simulink model "DSSDK_TrackerSingleObject"  (Simulink 9.3)
settings: Solver=FixedStepDiscrete  StartTime=0.0  StopTime=inf  FixedStep=Ts  RelTol=1e-3  EnableMultiTasking=on
StopFcn:
  | save('viconData.mat','viconData')
undefined symbols (not defined in the file or in its folder): fdesignblkfcn, gcbh
libraries: simulink x5, parrotlib x2
settings Model: Creator=Ssubrama  LastModifiedBy=yahyaaba
settings DataIOCC: LimitDataPoints=on
settings OptimizationCC: ExpressionDepthLimit=2147483647  InitFltsAndDblsToZero=on
settings DebuggingCC: SolverPrmCheckMsg=warning  StateNameClashWarn=warning
settings GRTTargetCC: TargetFcnLib=ansi_tfl_tmw_new.mat  GeneratePreprocessorConditionals=Disable all
settings ConfigComp: CovSFcnEnable=off

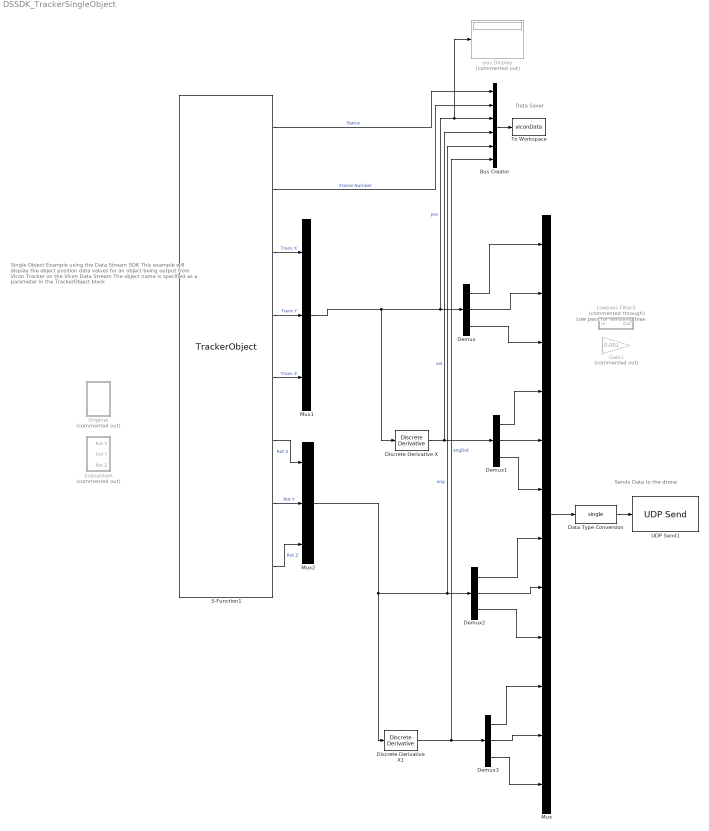
== system DSSDK_TrackerSingleObject ==
  note: Sends Data to the drone
  note: Data Saver
  note: Low pass for removing bias
  note: Single Object Example
      | using the Data Stream SDK
      |
      | This example will display the object position data
      | values for an object being output from
      | Vicon Tracker on the Vicon Data Stream
      |
      | The object name is specified as a parameter
      | in the TrackerObject block
  Bus Creator : BusCreator  Inputs=6
  Data Type Conversion : DataTypeConversion  OutDataTypeStr=single
  Demux{,1..3} (4 alike) : Demux  Outputs=3
  Discrete Derivative X : simulink/Discrete/Discrete Derivative  gainval=1.0  ICPrevScaledInput=0.0  OutMin=[]  OutMax=[]  OutDataType=fixdt(1, 16)  OutScaling=2^-10  DoSatur=off
  Discrete Derivative X1 : simulink/Discrete/Discrete Derivative  gainval=1.0  ICPrevScaledInput=0.0  OutMin=[]  OutMax=[]  OutDataType=fixdt(1, 16)  OutScaling=2^-10  DoSatur=off
  Gain1 : Gain  Commented=on  Gain=0.001
  Lowpass Filter3 : Subsystem  Commented=through  DialogController=fdesignblkfcn  DialogControllerArgs=DataTag1  InitFcn=fdesignblkfcn(gcbh, {'InitFcn'});  mask(Lowpass Filter){}
      mask help: Design a lowpass filter
      settings: CopyFcn=fdesignblkfcn(gcbh, {'CopyFcn'});
      mask Help: helpview(mapfilelocation('dsp'), 'dsplowpassfilter');
      mask Display: disp('Lowpass')
  Mux : Mux  Inputs=12
  Mux1 : Mux  Inputs=3
  Mux2 : Mux  Inputs=3
  Original : Subsystem  Commented=on
  S-Function1 : S-Function  FunctionName=TrackerObject  Parameters='ParrotMambo'  SFunctionModules=TrackerObject  SFunctionDeploymentMode=off  EnableBusSupport=off
      settings: AttributesFormatString=Data Parser
  Subsystem : Subsystem  Commented=on
  To Workspace : ToWorkspace  VariableName=viconData  SaveFormat=Timeseries  SampleTime=-1
  UDP Send1 : parrotlib/UDP Send  remoteURL='192.168.3.1'  remotePort=25000  localURL='0.0.0.0'  localPortSource=Automatically determine  localPort=2048  sampletime=-1  blockPlatform=LINUX  separateLengthPort=0
      settings: SourceProductName=Simulink Support Package for PARROT Minidrones  SourceProductBaseCode=MINIDRONES
  pos Display : Display  Commented=on
  wires:
  S-Function1/3 -> Mux1/1  "Trans X"
  S-Function1/5 -> Mux1/3  "Trans Z"
  Data Type Conversion/1 -> UDP Send1/1
  Mux/1 -> Data Type Conversion/1
  S-Function1/6 -> Mux2/1  "Rot X"
  S-Function1/7 -> Mux2/2  "Rot Y"
  S-Function1/8 -> Mux2/3  "Rot Z"
  S-Function1/1 -> Bus Creator/1  "Status"
  S-Function1/2 -> Bus Creator/2  "Frame Number"
  S-Function1/4 -> Mux1/2  "Trans Y"
  Mux1/1 -> pos Display/1, Bus Creator/3, Demux/1, Discrete Derivative X/1  "pos"
  Demux/1 -> Mux/1
  Demux/2 -> Mux/2
  Demux/3 -> Mux/3
  Demux1/1 -> Mux/4
  Demux1/2 -> Mux/5
  Demux1/3 -> Mux/6
  Demux2/1 -> Mux/7
  Demux2/2 -> Mux/8
  Demux2/3 -> Mux/9
  Discrete Derivative X1/1 -> Demux3/1, Bus Creator/6  "angDot"
  Demux3/1 -> Mux/10
  Demux3/2 -> Mux/11
  Demux3/3 -> Mux/12
  Mux2/1 -> Demux2/1, Bus Creator/5, Discrete Derivative X1/1  "ang"
  Discrete Derivative X/1 -> Bus Creator/4, Demux1/1  "vel"
  Bus Creator/1 -> To Workspace/1

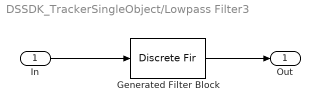
== system DSSDK_TrackerSingleObject/Lowpass Filter3 ==
  In : Inport
  Generated Filter Block : DiscreteFir  Tag=BlockMethodSubSystem  Coefficients=[0.00055930462501575318 0.000134387355635492544 0.000150164544220283578 0.000166938571918249026 0.000184913426126165478 0.000204159638341897876 0.000224847539957342317 0.000246888557047488118 0.000270250930713089371 0.000294678714756113928 0.000320320592567133189 0.000347381610550177703 0.000376503237496001526 0.000407063236803795311 0.000437969836956363285 0.000471966634088865277 0.000506629618629239609 0.000543258400010798704 0.000581446667477806102 0.000621483478831086908 0.000663240114968196475 0.000706786791731873467 0.000751966629339840078 0.000798957232007100585 0.000847786970567231948 0.000898567434806632503 0.000950986800426248521 0.00100536098241037187 0.00106189549677395854 0.00111999258611391694 0.00118025266269442377 0.00124231961860752629 0.00130642002474549318 0.00137244110948316739 0.00144041400814671496 0.00151028782591035434 0.00158214490911966644 0.00165593031316057463 0.00173161625085798245 0.00180913894205901355 0.00188869079631055563 0.00197008991505943183 0.00205326044396706353 0.00213839755526306231 0.00222523410058983809 0.0023139366140836953 0.00240433500877287442 0.00249647034146493986 0.00259028150327670834 0.00268577672918223105 0.00278284271081329342 0.00288145055032864748 0.00298156134317205564 0.00308318312494121945 0.0031861164566033065 0.00329041971903219245 0.00339602350822430007 0.00350278519574314436 0.00361074370565326631 0.00371971960476352465 0.00382972885080347814 0.00394066786669221118 0.00405247698115740549 0.00416504159927491568 0.00427831667671187306 0.00439222319691515498 0.00450666349417792877 0.00462150504328727105 0.00473675818605371994 0.0048522536812996564 0.00496792387820703223 0.00508369550725730566 0.00519941524626886878 0.00531505864840853791 0.00543047442906128414 0.00554558136902359722 0.00566026462488985246 0.00577445307225213627 0.00588802605681441188 0.00600086635173012646 0.00611287829882902096 0.00622399830399815272 0.00633405571686646452 0.00644301018993313247 0.00655072347056720461 0.00665709789858928702 0.00676205989040209836 0.00686546177223198301 0.00696722908918023624 0.00706725534584395215 0.00716545349111825242 0.00726170727371388321 0.00735591743291842421 0.00744801050560451022 0.00753788345848689558 0.0076254188763999961 0.00771057173373233817 0.00779320792465807571 0.00787327807504492778 0.00795068643545090992 0.00802533165362758101 0.00809716296896351162 0.00816609203546844568 0.00823205161182060871 0.00829495997208222306 0.00835475861758848935 0.00841139903382095468 0.00846479300015721449 0.00851489303009545818 0.0085616579958750251 0.00860500810577487923 0.0086449345827915719 0.00868135979237836738 0.00871425404479079894 0.00874359520388623412 0.00876933590254826839 0.00879145283398880331 0.00880991471525752537 0.00882471405033441632 0.00883583717884927483 0.0088432445604231108 0.00884695935983879043 0.00884695935983879043 0.0088432445604231108 0.00883583717884927483 0.00882471405033441632 0.00880991471525752537 0.00879145283398880331 0.00876933590254826839 0.00874359520388623412 0.00871425404479079894 0.00868135979237836738 0.0086449345827915719 0.00860500810577487923 0.0085616579958750251 0.00851489303009545818 0.00846479300015721449 0.00841139903382095468 0.00835475861758848935 0.00829495997208222306 0.00823205161182060871 0.00816609203546844568 0.00809716296896351162 0.00802533165362758101 0.00795068643545090992 0.00787327807504492778 0.00779320792465807571 0.00771057173373233817 0.0076254188763999961 0.00753788345848689558 0.00744801050560451022 0.00735591743291842421 0.00726170727371388321 0.00716545349111825242 0.00706725534584395215 0.00696722908918023624 0.00686546177223198301 0.00676205989040209836 0.00665709789858928702 0.00655072347056720461 0.00644301018993313247 0.00633405571686646452 0.00622399830399815272 0.00611287829882902096 0.00600086635173012646 0.00588802605681441188 0.00577445307225213627 0.00566026462488985246 0.00554558136902359722 0.00543047442906128414 0.00531505864840853791 0.00519941524626886878 0.00508369550725730566 ...(+1656 chars)]  InputProcessing=Columns as channels (frame based)
  Out : Outport
  wires:
  Generated Filter Block/1 -> Out/1
  In/1 -> Generated Filter Block/1

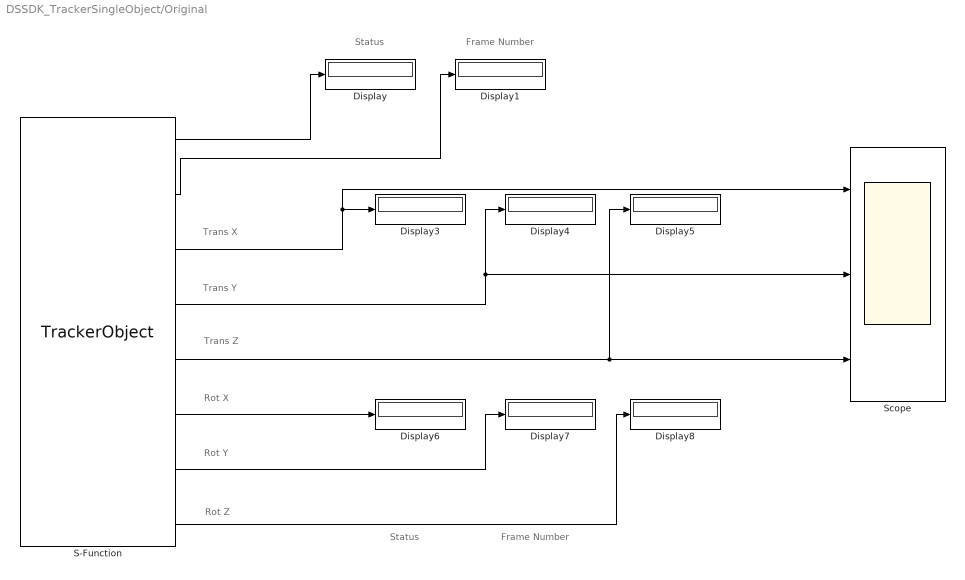
== system DSSDK_TrackerSingleObject/Original ==
  note: Rot Z
  note: Rot Y
  note: Rot X
  note: Trans Z
  note: Trans Y
  note: Trans X
  note: Frame Number
  note: Status
  note: Frame Number
  note: Status
  Display{,1,3..8} (8 alike) : Display
  S-Function : S-Function  FunctionName=TrackerObject  Parameters='Object1'  SFunctionModules=TrackerObject  SFunctionDeploymentMode=off  EnableBusSupport=off
      settings: AttributesFormatString=Data Parser
  Scope : Scope  NumInputPorts=3
  wires:
  S-Function/6 -> Display6/1
  S-Function/7 -> Display7/1
  S-Function/1 -> Display/1
  S-Function/4 -> Display4/1, Scope/2
  S-Function/8 -> Display8/1
  S-Function/5 -> Display5/1, Scope/3
  S-Function/2 -> Display1/1
  S-Function/3 -> Scope/1, Display3/1

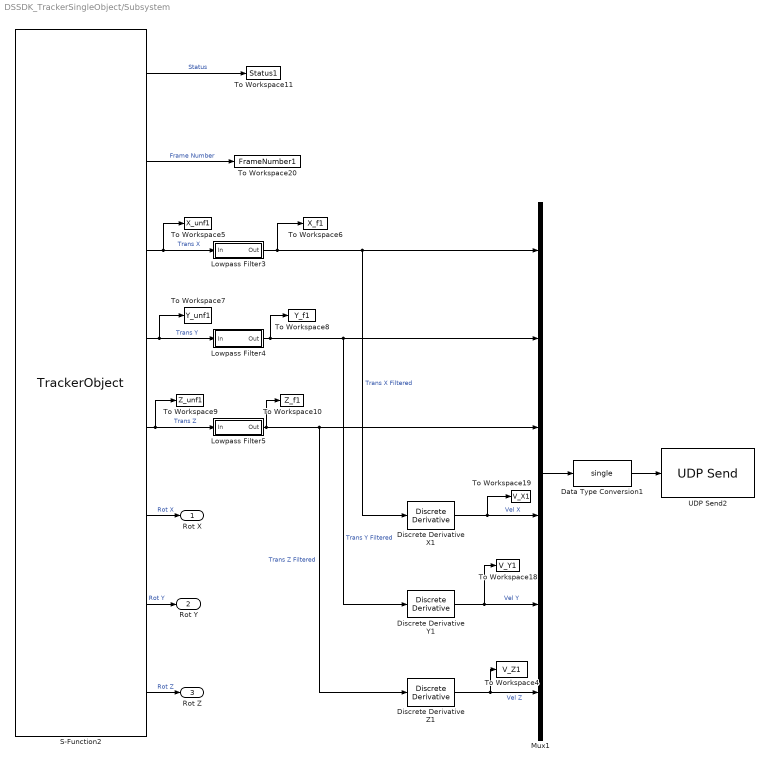
== system DSSDK_TrackerSingleObject/Subsystem ==
  Data Type Conversion1 : DataTypeConversion  OutDataTypeStr=single
  Discrete Derivative X1 : simulink/Discrete/Discrete Derivative  gainval=1.0  ICPrevScaledInput=0.0  OutMin=[]  OutMax=[]  OutDataType=fixdt(1, 16)  OutScaling=2^-10  DoSatur=off
  Discrete Derivative Y1 : simulink/Discrete/Discrete Derivative  gainval=1.0  ICPrevScaledInput=0.0  OutMin=[]  OutMax=[]  OutDataType=fixdt(1, 16)  OutScaling=2^-10  DoSatur=off
  Discrete Derivative Z1 : simulink/Discrete/Discrete Derivative  gainval=1.0  ICPrevScaledInput=0.0  OutMin=[]  OutMax=[]  OutDataType=fixdt(1, 16)  OutScaling=2^-10  DoSatur=off
  Lowpass Filter3 : Subsystem  DialogController=fdesignblkfcn  DialogControllerArgs=DataTag3  InitFcn=fdesignblkfcn(gcbh, {'InitFcn'});  mask(Lowpass Filter){}
      mask help: Design a lowpass filter
      settings: CopyFcn=fdesignblkfcn(gcbh, {'CopyFcn'});
      mask Help: helpview(mapfilelocation('dsp'), 'dsplowpassfilter');
      mask Display: disp('Lowpass')
  Lowpass Filter4 : Subsystem  DialogController=fdesignblkfcn  DialogControllerArgs=DataTag5  InitFcn=fdesignblkfcn(gcbh, {'InitFcn'});  mask(Lowpass Filter){}
      mask help: Design a lowpass filter
      settings: CopyFcn=fdesignblkfcn(gcbh, {'CopyFcn'});
      mask Help: helpview(mapfilelocation('dsp'), 'dsplowpassfilter');
      mask Display: disp('Lowpass')
  Lowpass Filter5 : Subsystem  DialogController=fdesignblkfcn  DialogControllerArgs=DataTag7  InitFcn=fdesignblkfcn(gcbh, {'InitFcn'});  mask(Lowpass Filter){}
      mask help: Design a lowpass filter
      settings: CopyFcn=fdesignblkfcn(gcbh, {'CopyFcn'});
      mask Help: helpview(mapfilelocation('dsp'), 'dsplowpassfilter');
      mask Display: disp('Lowpass')
  Mux1 : Mux  Inputs=6
  S-Function2 : S-Function  FunctionName=TrackerObject  Parameters='Object1'  SFunctionModules=TrackerObject  SFunctionDeploymentMode=off  EnableBusSupport=off
      settings: AttributesFormatString=Data Parser
  To Workspace10 : ToWorkspace  VariableName=Z_f1  SaveFormat=Timeseries  SampleTime=-1
  To Workspace11 : ToWorkspace  VariableName=Status1  SaveFormat=Timeseries  SampleTime=-1
  To Workspace18 : ToWorkspace  VariableName=V_Y1  SaveFormat=Timeseries  SampleTime=-1
  To Workspace19 : ToWorkspace  VariableName=V_X1  SaveFormat=Timeseries  SampleTime=-1
  To Workspace20 : ToWorkspace  VariableName=FrameNumber1  SaveFormat=Timeseries  SampleTime=-1
  To Workspace4 : ToWorkspace  VariableName=V_Z1  SaveFormat=Timeseries  SampleTime=-1
  To Workspace5 : ToWorkspace  VariableName=X_unf1  SaveFormat=Timeseries  SampleTime=-1
  To Workspace6 : ToWorkspace  VariableName=X_f1  SaveFormat=Timeseries  SampleTime=-1
  To Workspace7 : ToWorkspace  VariableName=Y_unf1  SaveFormat=Timeseries  SampleTime=-1
  To Workspace8 : ToWorkspace  VariableName=Y_f1  SaveFormat=Timeseries  SampleTime=-1
  To Workspace9 : ToWorkspace  VariableName=Z_unf1  SaveFormat=Timeseries  SampleTime=-1
  UDP Send2 : parrotlib/UDP Send  remoteURL='192.168.3.1'  remotePort=25000  localURL='0.0.0.0'  localPortSource=Automatically determine  localPort=2048  sampletime=-1  blockPlatform=LINUX  separateLengthPort=0
      settings: SourceProductName=Simulink Support Package for PARROT Minidrones  SourceProductBaseCode=MINIDRONES
  Rot X : Outport
  Rot Y : Outport  Port=2
  Rot Z : Outport  Port=3
  wires:
  S-Function2/7 -> Rot Y/1  "Rot Y"
  Lowpass Filter4/1(Out) -> Discrete Derivative Y1/1, Mux1/2, To Workspace8/1  "Trans Y Filtered"
  Discrete Derivative X1/1 -> Mux1/4, To Workspace19/1  "Vel X"
  S-Function2/5 -> Lowpass Filter5/1(In), To Workspace9/1  "Trans Z"
  S-Function2/4 -> Lowpass Filter4/1(In), To Workspace7/1  "Trans Y"
  S-Function2/2 -> To Workspace20/1  "Frame Number"
  Lowpass Filter5/1(Out) -> To Workspace10/1, Discrete Derivative Z1/1, Mux1/3  "Trans Z Filtered"
  Discrete Derivative Y1/1 -> To Workspace18/1, Mux1/5  "Vel Y"
  S-Function2/1 -> To Workspace11/1  "Status"
  Discrete Derivative Z1/1 -> To Workspace4/1, Mux1/6  "Vel Z"
  Mux1/1 -> Data Type Conversion1/1
  Data Type Conversion1/1 -> UDP Send2/1
  S-Function2/3 -> To Workspace5/1, Lowpass Filter3/1(In)  "Trans X"
  Lowpass Filter3/1(Out) -> Discrete Derivative X1/1, Mux1/1, To Workspace6/1  "Trans X Filtered"
  S-Function2/6 -> Rot X/1  "Rot X"
  S-Function2/8 -> Rot Z/1  "Rot Z"

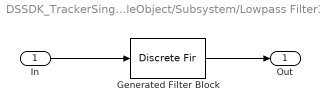
== system DSSDK_TrackerSingleObject/Subsystem/Lowpass Filter3 ==
  In : Inport
  Generated Filter Block : DiscreteFir  Tag=BlockMethodSubSystem  Coefficients=[0.000559304625015753397 0.000134387355635494116 0.000150164544220285801 0.00016693857191824946 0.000184913426126165478 0.00020415963834189831 0.000224847539957342317 0.000246888557047488118 0.000270250930713089588 0.0002946787147561155 0.000320320592567135195 0.000347381610550178842 0.000376503237496001472 0.000407063236803794769 0.000437969836956363719 0.000471966634088866199 0.000506629618629240042 0.000543258400010799571 0.00058144666747780762 0.000621483478831088101 0.000663240114968196908 0.000706786791731873034 0.000751966629339840295 0.000798957232007101669 0.00084778697056723184 0.000898567434806632395 0.000950986800426249172 0.00100536098241037252 0.00106189549677395919 0.00111999258611391803 0.00118025266269442442 0.00124231961860752672 0.00130642002474549426 0.00137244110948316826 0.00144041400814671539 0.00151028782591035478 0.001582144909119666 0.00165593031316057463 0.00173161625085798375 0.00180913894205901441 0.00188869079631055628 0.00197008991505943226 0.00205326044396706439 0.00213839755526306317 0.00222523410058983852 0.0023139366140836953 0.00240433500877287485 0.00249647034146493986 0.00259028150327670877 0.00268577672918223148 0.00278284271081329429 0.00288145055032864791 0.00298156134317205564 0.00308318312494121989 0.0031861164566033065 0.00329041971903219245 0.00339602350822430007 0.00350278519574314436 0.00361074370565326631 0.00371971960476352422 0.00382972885080347814 0.00394066786669221118 0.00405247698115740549 0.00416504159927491568 0.00427831667671187306 0.00439222319691515584 0.00450666349417792877 0.00462150504328727105 0.00473675818605371994 0.0048522536812996564 0.00496792387820703223 0.00508369550725730566 0.00519941524626886878 0.00531505864840853878 0.005430474429061285 0.00554558136902359722 0.00566026462488985246 0.00577445307225213627 0.00588802605681441188 0.00600086635173012646 0.00611287829882902096 0.00622399830399815186 0.00633405571686646365 0.00644301018993313161 0.00655072347056720548 0.00665709789858928702 0.00676205989040209836 0.00686546177223198127 0.00696722908918023538 0.00706725534584395128 0.00716545349111825242 0.00726170727371388321 0.00735591743291842334 0.00744801050560450935 0.00753788345848689471 0.0076254188763999961 0.00771057173373233731 0.00779320792465807398 0.00787327807504492605 0.00795068643545090818 0.00802533165362757928 0.00809716296896350989 0.00816609203546844395 0.00823205161182060698 0.00829495997208222133 0.00835475861758848762 0.00841139903382095294 0.00846479300015721275 0.00851489303009545818 0.0085616579958750251 0.00860500810577487923 0.0086449345827915719 0.00868135979237836738 0.00871425404479079721 0.00874359520388623065 0.00876933590254826839 0.00879145283398879984 0.00880991471525751843 0.00882471405033441458 0.00883583717884927136 0.00884324456042310733 0.0088469593598387887 0.0088469593598387887 0.00884324456042310733 0.00883583717884927136 0.00882471405033441458 0.00880991471525751843 0.00879145283398879984 0.00876933590254826839 0.00874359520388623065 0.00871425404479079721 0.00868135979237836738 0.0086449345827915719 0.00860500810577487923 0.0085616579958750251 0.00851489303009545818 0.00846479300015721275 0.00841139903382095294 0.00835475861758848762 0.00829495997208222133 0.00823205161182060698 0.00816609203546844395 0.00809716296896350989 0.00802533165362757928 0.00795068643545090818 0.00787327807504492605 0.00779320792465807398 0.00771057173373233731 0.0076254188763999961 0.00753788345848689471 0.00744801050560450935 0.00735591743291842334 0.00726170727371388321 0.00716545349111825242 0.00706725534584395128 0.00696722908918023538 0.00686546177223198127 0.00676205989040209836 0.00665709789858928702 0.00655072347056720548 0.00644301018993313161 0.00633405571686646365 0.00622399830399815186 0.00611287829882902096 0.00600086635173012646 0.00588802605681441188 0.00577445307225213627 0.00566026462488985246 0.00554558136902359722 0.005430474429061285 0.00531505864840853878 0.00519941524626886878 0.00508369550725730566 ...(+1649 chars)]  InputProcessing=Columns as channels (frame based)
  Out : Outport
  wires:
  Generated Filter Block/1 -> Out/1
  In/1 -> Generated Filter Block/1

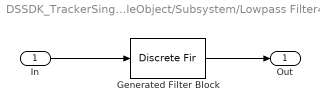
== system DSSDK_TrackerSingleObject/Subsystem/Lowpass Filter4 ==
  In : Inport
  Generated Filter Block : DiscreteFir  Tag=BlockMethodSubSystem  Coefficients=[-0.00084475613175170818 1.9130153688269205e-05 2.0214131432315304e-05 2.1928029829354306e-05 2.4591858738332392e-05 2.7878622988662786e-05 3.2100156662285447e-05 3.6940303166599174e-05 4.2729969430913146e-05 4.9143314424989633e-05 5.6520563576693486e-05 6.4545533413592538e-05 7.3571517288272104e-05 8.3254688671381856e-05 9.3941922219367835e-05 0.00010534594669243068 0.00011780449047032596 0.00013096794104900143 0.00014525080846465319 0.00016028645933404204 0.00017646269948090235 0.00019342002126192381 0.00021160729603197307 0.00023058415946953592 0.00025084901215922608 0.00027191751714601312 0.00029437012506591527 0.00031761443557428771 0.00034235870055102373 0.00036783395721458236 0.00039502995575715097 0.00042255042896937006 0.0004518767762923991 0.00048418773030947649 0.00051494100809876275 0.00054804427989728853 0.00058213756218483681 0.00061784798315962655 0.00065471827305482928 0.00069306960413741407 0.00073268232761762358 0.00077372135005837758 0.00081609069746628189 0.00085987316503132968 0.00090503058209321838 0.00095156551328557011 0.00099951546818382751 0.001048892608257861 0.0010996728696636513 0.0011518531722417306 0.0012055015205849687 0.0012605253652633679 0.0013170110985270323 0.0013748814670609161 0.0014342292385452677 0.0014949162566170874 0.0015570882439231736 0.0016205791230290594 0.0016855629877502753 0.0017518110149012918 0.0018195615332199763 0.0018885122556354917 0.0019589932401155178 0.0020304857282480568 0.0021037769014525818 0.0021780809180233706 0.0022532033797941289 0.0023300764047560697 0.002408019136506376 0.0024872548308788127 0.0025675724927420509 0.0026490658254767325 0.0027316187670979935 0.0028152502306164374 0.0028999040138936419 0.0029855467479533273 0.0030721437562002806 0.0031596300441931848 0.0032480499708169006 0.0033372864419940786 0.0034272961291024195 0.0035180686103771725 0.0036095579990111323 0.0037016684075071105 0.0037944135684569395 0.0038876930607518608 0.0039814964276640866 0.004075711319748535 0.0041703660467547849 0.0042653206053666556 0.0043606048584123921 0.0044560567980269934 0.0045517449946426139 0.0046474690456441269 0.0047433220000064023 0.0048390514628438921 0.0049349409920054453 0.0050303599695821393 0.005125736595535545 0.0052209974723502455 0.0053158489890522886 0.0054103178039552891 0.0055043205657833117 0.0055978063251341924 0.005690716277565842 0.0057829693413471136 0.0058745343201712331 0.0059652981406936589 0.0060552512421996251 0.0061442804836209716 0.0062324255936591928 0.0063194439869470823 0.0064053997566050009 0.0064902080815222229 0.0065737893569911762 0.0066560643832651364 0.0067370215675464501 0.0068165448230662201 0.0068946139509815183 0.0069711333227454025 0.0070460960482252701 0.0071193815044052157 0.0071909886035725675 0.0072608058816287686 0.0073288500361475941 0.0073949837462685295 0.0074592372551665455 0.0075214871224524851 0.0075817908735233185 0.0076398465235371187 0.0076960193405338625 0.007749943492233664 0.0078016385772204976 0.0078510611899593914 0.0078982280680865644 0.007943044994299377 0.0079855298083864566 0.0080255928298220078 0.0080632614601325366 0.0080984370778125949 0.0081311701259260336 0.0081613666291623348 0.0081890712340489443 0.0082140625713304511 0.0082366057814709671 0.0082564961260276088 0.0082737716511510906 0.0082883995318900217 0.0083004112324183491 0.0083097353618941973 0.0083164213144566266 0.0083204210874554211 0.0083217726939814676 0.0083204210874554211 0.0083164213144566266 0.0083097353618941973 0.0083004112324183491 0.0082883995318900217 0.0082737716511510906 0.0082564961260276088 0.0082366057814709671 0.0082140625713304511 0.0081890712340489443 0.0081613666291623348 0.0081311701259260336 0.0080984370778125949 0.0080632614601325366 0.0080255928298220078 0.0079855298083864566 0.007943044994299377 0.0078982280680865644 0.0078510611899593914 0.0078016385772204976 0.007749943492233664 0.0076960193405338625 0.0076398465235371187 0.0075817908735233185 0.0075214871224524851 0.0074592372551665455 0.0073949837462685295 ...(+2792 chars)]  InputProcessing=Columns as channels (frame based)
  Out : Outport
  wires:
  Generated Filter Block/1 -> Out/1
  In/1 -> Generated Filter Block/1

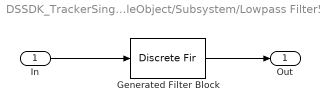
== system DSSDK_TrackerSingleObject/Subsystem/Lowpass Filter5 ==
  In : Inport
  Generated Filter Block : DiscreteFir  Tag=BlockMethodSubSystem  Coefficients=[0.0010438901225940831 0.00012354088148469351 0.00013070400115602399 0.00013834960280678036 0.00014596894146551005 0.00015403893168281359 0.00016203788292356918 0.00017055350569484217 0.00017907272657582301 0.00018831462117422986 0.00019765090346090652 0.00020784032141500067 0.00021767613324712772 0.00022794168442264817 0.00023659510580732745 0.00024880763191149631 0.00025982277257009573 0.00027040920537772014 0.00028234139711577643 0.00029386124097289601 0.00030624165518130771 0.00031856492905945753 0.00033157294629216011 0.0003445681564084828 0.00035808157890128824 0.00037157915937724819 0.00038570725102277613 0.00040003603069277448 0.0004150893606755414 0.00042970531424921926 0.00044493966348178318 0.00046085727937534454 0.00047660737867372084 0.00049301498023465566 0.00050956455082891157 0.0005265169938793332 0.00054372014428463397 0.00056130805099947521 0.0005792408532847165 0.00059756096394782338 0.0006161512503316352 0.00063502577047820619 0.00065421457556422537 0.0006739226870995439 0.00069396118060180445 0.00071404528982047509 0.0007348193050352688 0.00075568971982121623 0.00077700693244347444 0.00079863279711671017 0.00082062238264760307 0.00084292239903858816 0.00086553173206488181 0.00088844855846355233 0.00091173530528628702 0.00093537667142473268 0.00095932345213913678 0.00098351429226786052 0.0010080262831828227 0.0010330069942687532 0.0010581143509964313 0.0010836336364360136 0.001109463664928924 0.0011355293917327169 0.0011619534649647178 0.0011886280789465049 0.0012156698631213014 0.0012429654101590152 0.0012705580415228951 0.0012983830023958762 0.0013265479795755504 0.001354993647408586 0.0013837340640601783 0.0014126350481840399 0.0014419261003762306 0.0014714130799663582 0.0015011333695863142 0.0015311730914253831 0.0015614041068926483 0.0015919029258883212 0.0016225913209598534 0.0016535206600493311 0.0016846845100252006 0.0017160731807948006 0.0017476400685308582 0.0017793928875518793 0.0018113464482121318 0.0018435274156758802 0.0018758311748156844 0.001908318812522186 0.0019410202594715561 0.0019737934332837949 0.0020067752219371428 0.002039872015752607 0.0020731325612166384 0.0021065119403655846 0.0021399891885268527 0.0021735829551047673 0.0022072955644629215 0.0022411159135527774 0.0022750080964725602 0.0023089674681463935 0.0023430221050463888 0.0023771445752303164 0.0024112712791678433 0.0024455199876448684 0.0024797578031685147 0.0025140351181737065 0.0025483210653412343 0.0025826141369817597 0.0026169333177995069 0.0026512294580176106 0.0026854959299529913 0.0027197299895173649 0.0027539349518122393 0.0027880981426283221 0.0028221849623515875 0.0028562037711923017 0.00289017425063803 0.002924006033889807 0.00295775987972011 0.0029914204082208623 0.0030249432182058887 0.0030583585671591002 0.0030915958463266437 0.0031247114288090599 0.0031576658846565551 0.0031904568769100415 0.0032230561579368704 0.0032554700040130506 0.0032876899050400055 0.0033197046388299609 0.0033514760356486398 0.0033830587602360516 0.0034143897209073628 0.0034454509630193518 0.0034762784604740428 0.0035068197614344736 0.0035371132038200023 0.0035671004556680373 0.003596785990705815 0.0036261729309091544 0.0036552450425178747 0.0036839934327410301 0.0037124021185351544 0.0037404679590860787 0.0037681950789115858 0.0037955321897746325 0.0038225051511365576 0.0038491223019023321 0.0038753262227017014 0.0039011429505233105 0.003926538886960422 0.0039515250460640658 0.0039761051326994666 0.0040002299223065741 0.0040239296135573714 0.004047169367580164 0.0040699648417800646 0.0040922859863476921 0.00411413656626678 0.0041355187713854654 0.0041564202711735047 0.0041767935359899502 0.0041966996825622705 0.0042160831749616951 0.0042349667294033985 0.0042533205776213228 0.0042711382044104528 0.004288437491282584 0.0043051923386315423 0.0043213986168101921 0.0043370622014110875 0.0043521611884634517 0.0043667118550219566 0.0043806727294754735 0.0043940731400972117 0.004406912910723584 0.0044191576567501056 0.0044308100349050574 ...(+4780 chars)]  InputProcessing=Columns as channels (frame based)
  Out : Outport
  wires:
  Generated Filter Block/1 -> Out/1
  In/1 -> Generated Filter Block/1
